simulink model "FDMA_simTxRx_2020"  (R2016a)
settings: Solver=ode45  StartTime=0.0  StopTime=20  MaxStep=.01  MinStep=.001  RelTol=1e-3
libraries: dsparch4 x2
settings Model: Creator=user  LastModifiedBy=Simona
settings DataIOCC: LimitDataPoints=on  SaveFormat=Array  SignalLoggingSaveFormat=ModelDataLogs
settings OptimizationCC: ExpressionDepthLimit=2147483647  InitFltsAndDblsToZero=on
settings DebuggingCC: SaveWithParameterizedLinksMsg=none  UnderspecifiedInitializationDetection=Classic  MergeDetectMultiDrivingBlocksExec=none  SolverPrmCheckMsg=warning  MultiTaskCondExecSysMsg=none  FcnCallInpInsideContextMsg=UseLocalSettings  StateNameClashWarn=warning
settings HardwareCC: ProdBitPerPointer=32  ProdLargestAtomicFloat=None  ProdIntDivRoundTo=Undefined  ProdEndianess=Unspecified  ProdWordSize=32  ProdHWDeviceType=32-bit Generic
settings ModelReferenceCC: PropagateSignalLabelsOutOfModel=off
settings GRTTargetCC: CombineOutputUpdateFcns=off  GRTInterface=on
settings ConfigComp: CovModelRefEnable=Off

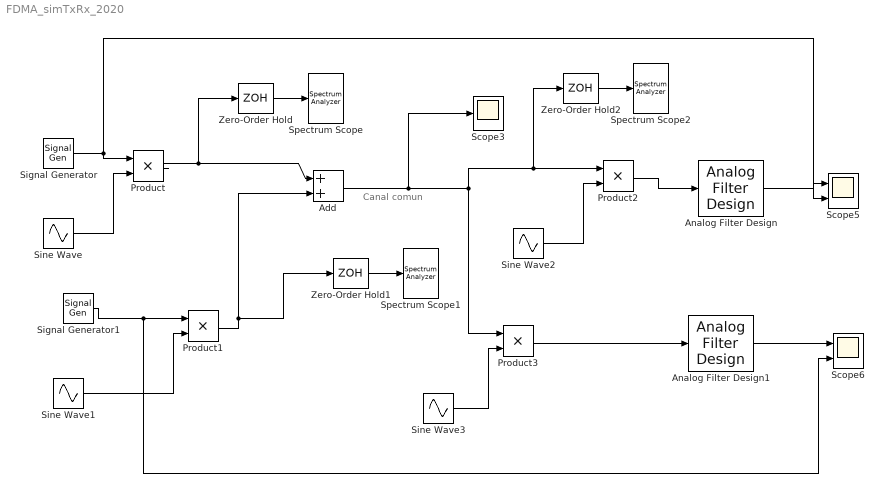
== system FDMA_simTxRx_2020 ==
  note: Canal comun
  Add : Sum
  Analog Filter Design : dsparch4/Analog Filter Design  method=Butterworth  filttype=Lowpass  N=10  Wlo=5*2*pi  Whi=80  Rp=2  Rs=40
  Analog Filter Design1 : dsparch4/Analog Filter Design  method=Butterworth  filttype=Lowpass  N=10  Wlo=5*2*pi  Whi=80  Rp=2  Rs=40
  Product{,1..3} (4 alike) : Product  RndMeth=Zero
  Scope3 : Scope
  Scope5 : Scope  NumInputPorts=2
  Scope6 : Scope  NumInputPorts=2
  Signal Generator : SignalGenerator
  Signal Generator1 : SignalGenerator  WaveForm=sawtooth  Frequency=2
  Sine Wave : Sin  Frequency=2*pi*10  SampleTime=0
  Sine Wave1 : Sin  Frequency=2*pi*20  SampleTime=0
  Sine Wave2 : Sin  Frequency=2*pi*10  SampleTime=0
  Sine Wave3 : Sin  Frequency=2*pi*20  SampleTime=0
  Spectrum Scope : SpectrumAnalyzer
  Spectrum Scope1 : SpectrumAnalyzer
  Spectrum Scope2 : SpectrumAnalyzer
  Zero-Order Hold : ZeroOrderHold  SampleTime=.01
  Zero-Order Hold1 : ZeroOrderHold  SampleTime=.01
  Zero-Order Hold2 : ZeroOrderHold  SampleTime=.01
  wires:
  Signal Generator/1 -> Product/1, Scope5/2
  Sine Wave/1 -> Product/2
  Product/1 -> Add/1, Zero-Order Hold/1
  Signal Generator1/1 -> Product1/1, Scope6/2
  Analog Filter Design/1 -> Scope5/1
  Analog Filter Design1/1 -> Scope6/1
  Sine Wave1/1 -> Product1/2
  Product1/1 -> Add/2, Zero-Order Hold1/1
  Sine Wave2/1 -> Product2/2
  Product2/1 -> Analog Filter Design/1
  Sine Wave3/1 -> Product3/2
  Product3/1 -> Analog Filter Design1/1
  Add/1 -> Scope3/1, Product2/1, Zero-Order Hold2/1, Product3/1
  Zero-Order Hold/1 -> Spectrum Scope/1
  Zero-Order Hold1/1 -> Spectrum Scope1/1
  Zero-Order Hold2/1 -> Spectrum Scope2/1
